simulink model "MASTER"  (R2018a)
settings: Solver=VariableStepAuto  StartTime=0.0  StopTime=inf  RelTol=1e-3
undefined symbols (not defined in the file): CR, LF, serial
libraries: instrumentlib x3, fuzblock x1
settings Model: Creator=helpe  LastModifiedBy=helpe

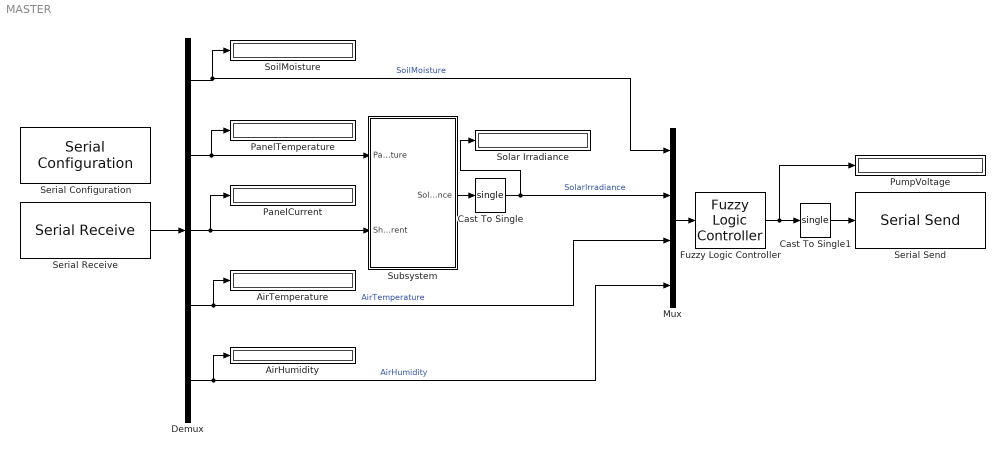
== system MASTER ==
  AirHumidity : Display
      settings: Format=decimal (Stored Integer)
  AirTemperature : Display
      settings: Format=decimal (Stored Integer)
  Cast To Single : DataTypeConversion  OutDataTypeStr=single
  Cast To Single1 : DataTypeConversion  OutDataTypeStr=single
  Demux : Demux  Outputs=5
  Fuzzy Logic Controller : fuzblock/Fuzzy Logic  Controller  FIS=PV2  OutputSampleNumber=101  DataType=double  FuzzifiedInputs=off  RuleFiringStrengths=off  RuleOutputs=off  AggregatedOutputs=off  SimulateUsing=Interpreted execution  OutOfRangeInputValueMessage=warning  NoRuleFiredMessage=warning  EmptyOutputFuzzySetMessage=warning
  Mux : Mux
  PanelCurrent : Display
      settings: Format=decimal (Stored Integer)
  PanelTemperature : Display
      settings: Format=decimal (Stored Integer)
  PumpVoltage : Display
      settings: Format=decimal (Stored Integer)
  Serial Configuration : instrumentlib/Serial Configuration  Priority=-200000  ComPortMenu=COM3  ComPort=COM3  ObjConstructor=serial('COM3');  BaudRate=9600  DataBits=8  Parity=none  StopBits=1  FlowControl=none  Timeout=10  ByteOrder=LittleEndian
  Serial Receive : instrumentlib/Serial Receive  ComPortMenu=COM3  ComPort=COM3  ObjConstructor=serial('COM3');  Terminator=CR/LF ('\r\n')  DataSize="[1  5]"  DataType=single  EnableBlockingMode=on  ActionDataUnavailable=Output last received value  CustomValue=0  SampleTime=0.01
  Serial Send : instrumentlib/Serial Send  ComPortMenu=COM3  ComPort=COM3  ObjConstructor=serial('COM3');  Terminator=CR/LF ('\r\n')  EnableBlockingMode=on
  SoilMoisture : Display
      settings: Format=decimal (Stored Integer)
  Solar Irradiance : Display
      settings: Format=decimal (Stored Integer)
  Subsystem : Subsystem
  wires:
  Serial Receive/1 -> Demux/1
  Demux/1 -> Mux/1, SoilMoisture/1  "SoilMoisture"
  Demux/4 -> AirTemperature/1, Mux/3  "AirTemperature"
  Demux/5 -> AirHumidity/1, Mux/4  "AirHumidity"
  Demux/2 -> PanelTemperature/1, Subsystem/1(Panel Temperature)
  Mux/1 -> Fuzzy Logic Controller/1
  Subsystem/1(Solar Irradiance) -> Cast To Single/1
  Fuzzy Logic Controller/1 -> Cast To Single1/1, PumpVoltage/1
  Cast To Single/1 -> Mux/2, Solar Irradiance/1  "SolarIrradiance"
  Cast To Single1/1 -> Serial Send/1
  Demux/3 -> Subsystem/2(Short Circuit Current), PanelCurrent/1

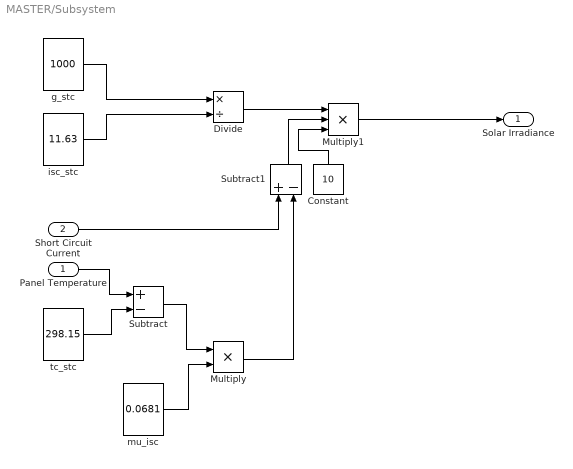
== system MASTER/Subsystem ==
  Panel Temperature : Inport
  Short Circuit Current : Inport  Port=2
  Constant : Constant  Value=10
  Divide : Product  Inputs=*/
  Multiply : Product
  Multiply1 : Product  Inputs=3
  Subtract : Sum  Inputs=+-
  Subtract1 : Sum  Inputs=+-
  g_stc : Constant  Value=1000
  isc_stc : Constant  Value=11.63
  mu_isc : Constant  Value=0.0681
  tc_stc : Constant  Value=298.15
  Solar Irradiance : Outport
  wires:
  g_stc/1 -> Divide/1
  isc_stc/1 -> Divide/2
  Panel Temperature/1 -> Subtract/1
  tc_stc/1 -> Subtract/2
  mu_isc/1 -> Multiply/2
  Subtract/1 -> Multiply/1
  Short Circuit Current/1 -> Subtract1/1
  Multiply/1 -> Subtract1/2
  Multiply1/1 -> Solar Irradiance/1
  Subtract1/1 -> Multiply1/2
  Divide/1 -> Multiply1/1
  Constant/1 -> Multiply1/3
